simulink model "lineFollowerModel"  (R2020a)
settings: Solver=ode4  StartTime=0.0  StopTime=5  FixedStep=0.0001  RelTol=1e-3
values from neighbouring files (symbols this model uses):
  b = -0.05    [define_constants.m]
  cRoll = 0.1    [define_constants.m]
  g = 9.81    [define_constants.m]
  I_T = 0.1    [define_constants.m]
  I_yy = 5.0000e-05    (= 5e-05)    [define_constants.m]
  K = 0.0089    [define_constants.m]
  L = 2.3E-2    (= 0.023)    [define_constants.m]
  m_T = 1 * mass_scale    [define_constants.m]
  N = 50    [define_constants.m]
  R = Orientation    [GeoVerMakeCyl.m]    (also in define_constants.m = 2.2)
  row1 = 0.1    [define_constants.m]
  row2 = row1*wheel_ratio_scale    [define_constants.m]
  sX = row1    (= 0.1)    [define_constants.m]
  sY = 0    [define_constants.m]
  Vmax = 12    [define_constants.m]
  W = line_width/2    [define_constants.m]
  xLp = [(xL(1) - padamount*gridsize):gridsize:xL(1)-gridsize, xL, xL(end)+gridsize:gridsize:xL(end)+padamount*gridsize]    [define_constants.m]
  yLp = [(yL(1) - padamount*gridsize):gridsize:yL(1)-gridsize, yL, yL(end)+gridsize:gridsize:yL(end)+padamount*gridsize]    [define_constants.m]
  Z = zeros(dims)    [define_constants.m]
libraries: simulink x10
settings Model: Creator=Amir  LastModifiedBy=matthewterblanche
settings SFSimCC: CustomCodeUndefinedFunction=UseInterfaceOnly

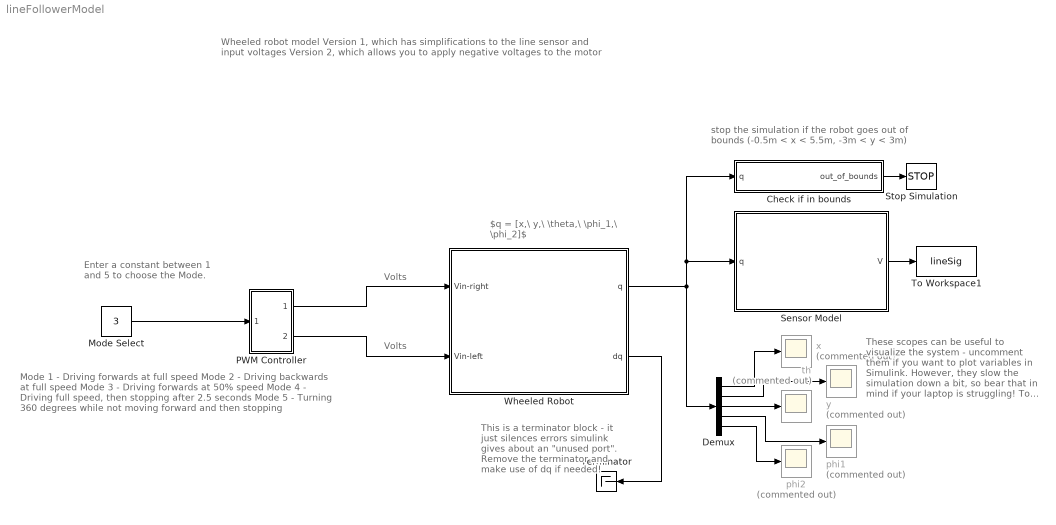
== system lineFollowerModel ==
  note: Volts
  note: stop the simulation if the robot goes out of bounds (-0.5m < x < 5.5m, -3m < y < 3m)
  note: Wheeled robot model
      | Version 1, which has simplifications to the line sensor and input voltages
      | Version 2, which allows you to apply negative voltages to the motor
  note: This is a terminator block - it just silences errors simulink gives about an "unused port". Remove the terminator and make use of dq if needed!
  note: These scopes can be useful to visualize the system - uncomment them if you want to plot variables in Simulink. However, they slow the simulation down a bit, so bear that in mind if your laptop is struggling!
      |
      | To make them work again, select the blocks > right click > Uncomment
  note: $q = [x,\ y,\ \theta,\ \phi_1,\ \phi_2]$
  note: Enter a constant between 1 and 5 to choose the Mode.
  note: Mode 1 - Driving forwards at full speed
      |
      | Mode 2 - Driving backwards at full speed
      |
      | Mode 3 - Driving forwards at 50% speed
      |
      | Mode 4 - Driving full speed, then stopping after 2.5 seconds
      |
      | Mode 5 - Turning 360 degrees while not moving forward and 			 then stopping
  note: Volts
  Check if in bounds : MATLAB Function  TreatAsAtomicUnit=on
  Demux : Demux  Outputs=5
  Mode Select : Constant  Value=3
  PWM Controller : Subsystem
  Sensor Model : Subsystem
  Stop Simulation : Stop
  Terminator : Terminator
  To Workspace1 : ToWorkspace  VariableName=lineSig  SampleTime=-1
  Wheeled Robot : Subsystem
  phi1 : Scope  Commented=on
  phi2 : Scope  Commented=on
  th : Scope  Commented=on
  x : Scope  Commented=on
  y : Scope  Commented=on
  wires:
  Demux/1 -> x/1
  Demux/2 -> y/1
  Demux/3 -> th/1
  Demux/4 -> phi1/1
  Demux/5 -> phi2/1
  Wheeled Robot/1(q) -> Sensor Model/1(q), Check if in bounds/1(q), Demux/1
  Sensor Model/1(V) -> To Workspace1/1
  Wheeled Robot/2(dq) -> Terminator/1
  Check if in bounds/1(out_of_bounds) -> Stop Simulation/1
  Mode Select/1 -> PWM Controller/1(In1)
  PWM Controller/1(Out1) -> Wheeled Robot/1(Vin-right)
  PWM Controller/2(Out2) -> Wheeled Robot/2(Vin-left)

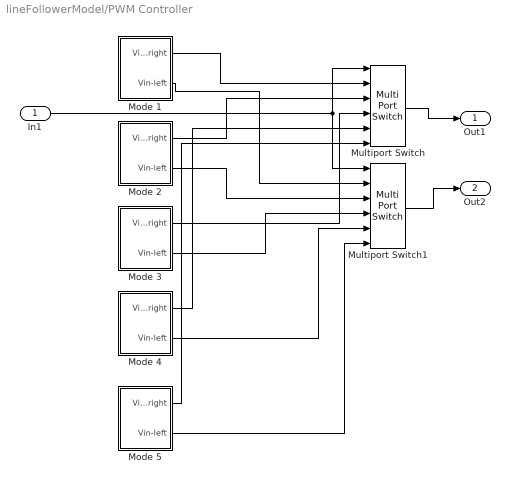
== system lineFollowerModel/PWM Controller ==
  In1 : Inport
  Mode 1 : Subsystem
  Mode 2 : Subsystem
  Mode 3 : Subsystem
  Mode 4 : Subsystem
  Mode 5 : Subsystem
  Multiport Switch : MultiPortSwitch  Inputs=5
  Multiport Switch1 : MultiPortSwitch  Inputs=5
  Out1 : Outport
  Out2 : Outport  Port=2
  wires:
  Multiport Switch/1 -> Out1/1
  Multiport Switch1/1 -> Out2/1
  In1/1 -> Multiport Switch/1, Multiport Switch1/1
  Mode 2/2(Vin-left) -> Multiport Switch1/3
  Mode 3/1(Vin-right) -> Multiport Switch/4
  Mode 5/2(Vin-left) -> Multiport Switch1/6
  Mode 4/1(Vin-right) -> Multiport Switch/5
  Mode 5/1(Vin-right) -> Multiport Switch/6
  Mode 2/1(Vin-right) -> Multiport Switch/3
  Mode 1/1(Vin-right) -> Multiport Switch/2
  Mode 1/2(Vin-left) -> Multiport Switch1/2
  Mode 4/2(Vin-left) -> Multiport Switch1/5
  Mode 3/2(Vin-left) -> Multiport Switch1/4

== system lineFollowerModel/Sensor Model ==
  q : Inport
  2-D Lookup Table : Lookup_n-D  BreakpointsForDimension1=xLp  BreakpointsForDimension2=yLp  Table=Z  InternalRulePriority=Speed  RndMeth=Simplest  InputSameDT=on
  MATLAB Function : MATLAB Function  TreatAsAtomicUnit=on
  V : Outport
  wires:
  MATLAB Function/1(posX) -> 2-D Lookup Table/1
  q/1 -> MATLAB Function/1(q)
  MATLAB Function/2(posY) -> 2-D Lookup Table/2
  2-D Lookup Table/1 -> V/1

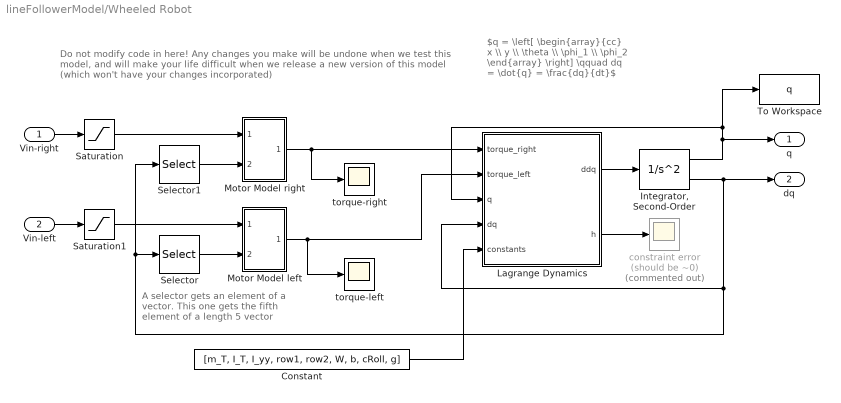
== system lineFollowerModel/Wheeled Robot ==
  note: A selector gets an element of a vector. This one gets the fifth element of a length 5 vector
  note: Do not modify code in here! Any changes you make will be undone when we test this model, and will make your life difficult when we release a new version of this model (which won't have your changes incorporated)
  note: $q = \left[ \begin{array}{cc} x \\ y \\ \theta \\ \phi_1 \\ \phi_2 \end{array} \right] \qquad dq = \dot{q} = \frac{dq}{dt}$
  Vin-right : Inport
  Vin-left : Inport  Port=2
  Constant : Constant  Value=[m_T, I_T, I_yy, row1, row2, W, b, cRoll, g]
  "Integrator, Second-Order" : SecondOrderIntegrator  ICX=[0 0 0 0 0]  ICDXDT=[0 0 0 0 0]
  Lagrange Dynamics : MATLAB Function  TreatAsAtomicUnit=on
  "Motor Model left " : Subsystem
  Motor Model right : Subsystem
  Saturation : Saturate  UpperLimit=Vmax  LowerLimit=-Vmax
  Saturation1 : Saturate  UpperLimit=Vmax  LowerLimit=-Vmax
  Selector : Selector  InputPortWidth=5  IndexOptions=Index vector (dialog)  Indices=[5]  OutputSizes=1
  Selector1 : Selector  InputPortWidth=5  IndexOptions=Index vector (dialog)  Indices=[4]  OutputSizes=1
  To Workspace : ToWorkspace  VariableName=q  SampleTime=0.01
  constraint error (should be ~0) : Scope  Commented=on
  torque-left : Scope
  torque-right : Scope
  q : Outport
  dq : Outport  Port=2
  wires:
  Selector/1 -> "Motor Model left "/2(Omega)
  Selector1/1 -> Motor Model right/2(Omega)
  Motor Model right/1(Tout) -> Lagrange Dynamics/1(torque_right), torque-right/1
  Vin-right/1 -> Saturation/1
  Vin-left/1 -> Saturation1/1
  "Integrator, Second-Order"/1 -> To Workspace/1, Lagrange Dynamics/3(q), q/1
  "Motor Model left "/1(Tout) -> Lagrange Dynamics/2(torque_left), torque-left/1
  "Integrator, Second-Order"/2 -> dq/1, Lagrange Dynamics/4(dq), Selector/1, Selector1/1
  Saturation/1 -> Motor Model right/1(Vin)
  Saturation1/1 -> "Motor Model left "/1(Vin)
  Lagrange Dynamics/1(ddq) -> "Integrator, Second-Order"/1
  Lagrange Dynamics/2(h) -> constraint error (should be ~0)/1
  Constant/1 -> Lagrange Dynamics/5(constants)

== system lineFollowerModel/PWM Controller/Mode 1 ==
  Subsystem : Subsystem
  Subsystem1 : Subsystem
  Vin-right : Outport
  Vin-left : Outport  Port=2
  wires:
  Subsystem1/1(Vin-left) -> Vin-left/1
  Subsystem/1(Vin-right) -> Vin-right/1

== system lineFollowerModel/PWM Controller/Mode 2 ==
  Subsystem : Subsystem
  Subsystem1 : Subsystem
  Vin-right : Outport
  Vin-left : Outport  Port=2
  wires:
  Subsystem1/1(Vin-left) -> Vin-left/1
  Subsystem/1(Vin-right) -> Vin-right/1

== system lineFollowerModel/PWM Controller/Mode 3 ==
  Subsystem : Subsystem
  Subsystem1 : Subsystem
  Vin-right : Outport
  Vin-left : Outport  Port=2
  wires:
  Subsystem1/1(Vin-left) -> Vin-left/1
  Subsystem/1(Vin-right) -> Vin-right/1

== system lineFollowerModel/PWM Controller/Mode 4 ==
  note: Stop motor after 2.5s
  Constant : Constant  Value=0
  Product : Product
  Product1 : Product
  Subsystem : Subsystem
  Subsystem1 : Subsystem
  Transport Delay : TransportDelay  DelayTime=2.5  InitialOutput=1  BufferSize=25600
  Vin-right : Outport
  Vin-left : Outport  Port=2
  wires:
  Subsystem1/1(Vin-left) -> Product/2
  Subsystem/1(Vin-right) -> Product1/2
  Product/1 -> Vin-left/1
  Product1/1 -> Vin-right/1
  Transport Delay/1 -> Product/1, Product1/1
  Constant/1 -> Transport Delay/1

== system lineFollowerModel/PWM Controller/Mode 5 ==
  Constant : Constant  Value=0
  Product : Product
  Product1 : Product
  Subsystem : Subsystem
  Subsystem1 : Subsystem
  Time motor must be on : TransportDelay  DelayTime=(0.175*pi/0.75)  InitialOutput=1  BufferSize=8192
  Vin-right : Outport
  Vin-left : Outport  Port=2
  wires:
  Constant/1 -> Time motor must be on/1
  Time motor must be on/1 -> Product1/1, Product/1
  Subsystem/1(Vin-right) -> Product/2
  Product/1 -> Vin-right/1
  Subsystem1/1(Vin-left) -> Product1/2
  Product1/1 -> Vin-left/1

== system lineFollowerModel/Wheeled Robot/Motor Model left  ==
  Vin : Inport
  Omega : Inport  Port=2
  Integrator : Integrator
  KT : Gain  Gain=K
  current dynamics : MATLAB Function  TreatAsAtomicUnit=on
  gear : Gain  Gain=N
  gear1 : Gain  Gain=N
  Tout : Outport  VectorParamsAs1DForOutWhenUnconnected=off
  wires:
  gear1/1 -> current dynamics/3(dth)
  Integrator/1 -> current dynamics/2(i), KT/1
  Omega/1 -> gear1/1
  gear/1 -> Tout/1
  current dynamics/1(di) -> Integrator/1
  KT/1 -> gear/1
  Vin/1 -> current dynamics/1(V)

== system lineFollowerModel/Wheeled Robot/Motor Model right ==
  Vin : Inport
  Omega : Inport  Port=2
  Integrator : Integrator
  KT : Gain  Gain=K
  current dynamics : MATLAB Function  TreatAsAtomicUnit=on
  gear : Gain  Gain=N
  gear1 : Gain  Gain=N
  Tout : Outport  VectorParamsAs1DForOutWhenUnconnected=off
  wires:
  Vin/1 -> current dynamics/1(V)
  KT/1 -> gear/1
  current dynamics/1(di) -> Integrator/1
  gear/1 -> Tout/1
  Omega/1 -> gear1/1
  Integrator/1 -> current dynamics/2(i), KT/1
  gear1/1 -> current dynamics/3(dth)

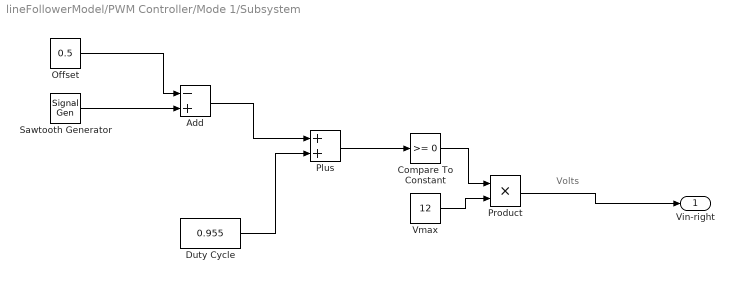
== system lineFollowerModel/PWM Controller/Mode 1/Subsystem ==
  note: Volts
  Add : Sum  Inputs=-+
  Compare To Constant : simulink/Logic and Bit Operations/Compare To Constant  relop=>=  const=0  OutDataTypeStr=boolean
  Duty Cycle : Constant  Value=0.955
  Offset : Constant  Value=0.5
  Plus : Sum
  Product : Product
  Sawtooth Generator : SignalGenerator  WaveForm=sawtooth  Amplitude=0.5  Frequency=10
  Vmax : Constant  Value=12
  Vin-right : Outport
  wires:
  Sawtooth Generator/1 -> Add/2
  Product/1 -> Vin-right/1
  Vmax/1 -> Product/2
  Duty Cycle/1 -> Plus/2
  Plus/1 -> Compare To Constant/1
  Offset/1 -> Add/1
  Compare To Constant/1 -> Product/1
  Add/1 -> Plus/1

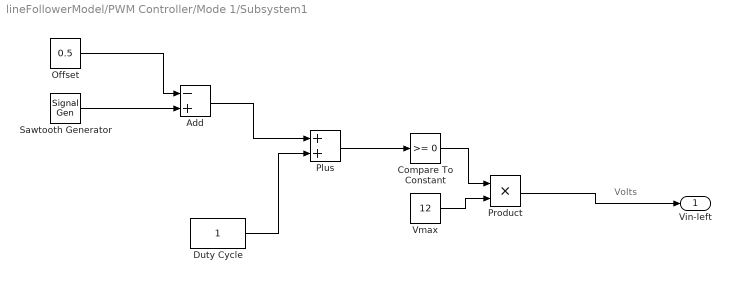
== system lineFollowerModel/PWM Controller/Mode 1/Subsystem1 ==
  note: Volts
  Add : Sum  Inputs=-+
  Compare To Constant : simulink/Logic and Bit Operations/Compare To Constant  relop=>=  const=0  OutDataTypeStr=boolean
  Duty Cycle : Constant
  Offset : Constant  Value=0.5
  Plus : Sum
  Product : Product
  Sawtooth Generator : SignalGenerator  WaveForm=sawtooth  Amplitude=0.5  Frequency=10
  Vmax : Constant  Value=12
  Vin-left : Outport
  wires:
  Sawtooth Generator/1 -> Add/2
  Product/1 -> Vin-left/1
  Vmax/1 -> Product/2
  Duty Cycle/1 -> Plus/2
  Plus/1 -> Compare To Constant/1
  Offset/1 -> Add/1
  Compare To Constant/1 -> Product/1
  Add/1 -> Plus/1

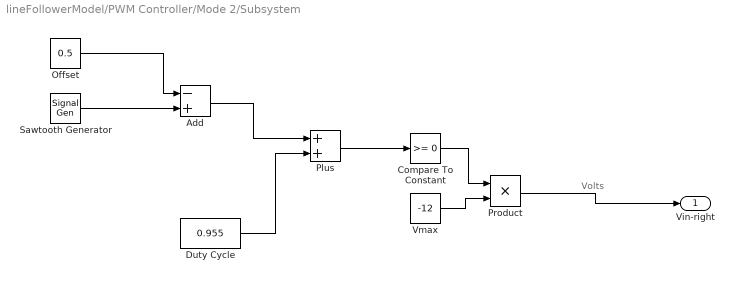
== system lineFollowerModel/PWM Controller/Mode 2/Subsystem ==
  note: Volts
  Add : Sum  Inputs=-+
  Compare To Constant : simulink/Logic and Bit Operations/Compare To Constant  relop=>=  const=0  OutDataTypeStr=boolean
  Duty Cycle : Constant  Value=0.955
  Offset : Constant  Value=0.5
  Plus : Sum
  Product : Product
  Sawtooth Generator : SignalGenerator  WaveForm=sawtooth  Amplitude=0.5  Frequency=10
  Vmax : Constant  Value=-12
  Vin-right : Outport
  wires:
  Sawtooth Generator/1 -> Add/2
  Product/1 -> Vin-right/1
  Vmax/1 -> Product/2
  Duty Cycle/1 -> Plus/2
  Plus/1 -> Compare To Constant/1
  Offset/1 -> Add/1
  Compare To Constant/1 -> Product/1
  Add/1 -> Plus/1

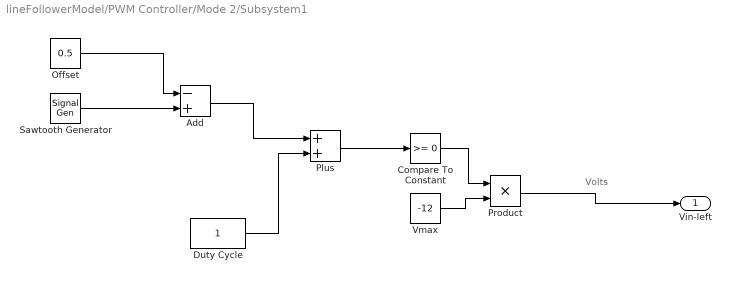
== system lineFollowerModel/PWM Controller/Mode 2/Subsystem1 ==
  note: Volts
  Add : Sum  Inputs=-+
  Compare To Constant : simulink/Logic and Bit Operations/Compare To Constant  relop=>=  const=0  OutDataTypeStr=boolean
  Duty Cycle : Constant
  Offset : Constant  Value=0.5
  Plus : Sum
  Product : Product
  Sawtooth Generator : SignalGenerator  WaveForm=sawtooth  Amplitude=0.5  Frequency=10
  Vmax : Constant  Value=-12
  Vin-left : Outport
  wires:
  Sawtooth Generator/1 -> Add/2
  Product/1 -> Vin-left/1
  Vmax/1 -> Product/2
  Duty Cycle/1 -> Plus/2
  Plus/1 -> Compare To Constant/1
  Offset/1 -> Add/1
  Compare To Constant/1 -> Product/1
  Add/1 -> Plus/1

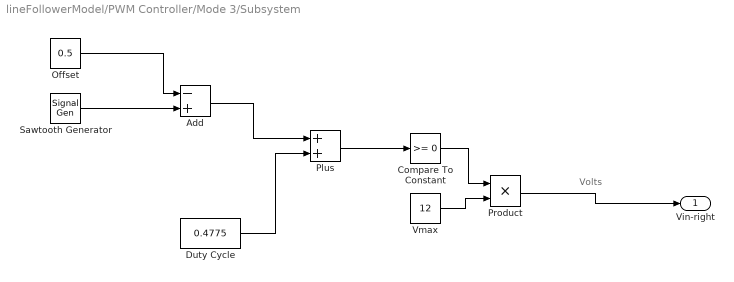
== system lineFollowerModel/PWM Controller/Mode 3/Subsystem ==
  note: Volts
  Add : Sum  Inputs=-+
  Compare To Constant : simulink/Logic and Bit Operations/Compare To Constant  relop=>=  const=0  OutDataTypeStr=boolean
  Duty Cycle : Constant  Value=0.4775
  Offset : Constant  Value=0.5
  Plus : Sum
  Product : Product
  Sawtooth Generator : SignalGenerator  WaveForm=sawtooth  Amplitude=0.5  Frequency=10
  Vmax : Constant  Value=12
  Vin-right : Outport
  wires:
  Sawtooth Generator/1 -> Add/2
  Product/1 -> Vin-right/1
  Vmax/1 -> Product/2
  Duty Cycle/1 -> Plus/2
  Plus/1 -> Compare To Constant/1
  Offset/1 -> Add/1
  Compare To Constant/1 -> Product/1
  Add/1 -> Plus/1

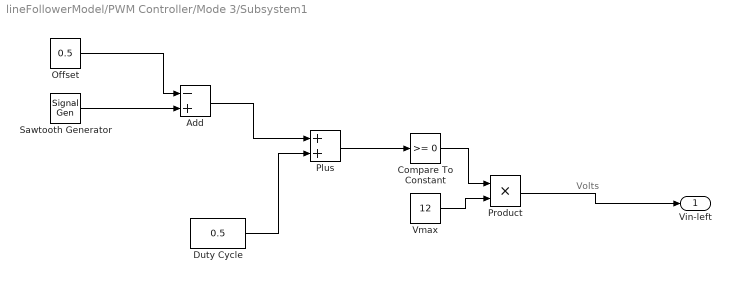
== system lineFollowerModel/PWM Controller/Mode 3/Subsystem1 ==
  note: Volts
  Add : Sum  Inputs=-+
  Compare To Constant : simulink/Logic and Bit Operations/Compare To Constant  relop=>=  const=0  OutDataTypeStr=boolean
  Duty Cycle : Constant  Value=0.5
  Offset : Constant  Value=0.5
  Plus : Sum
  Product : Product
  Sawtooth Generator : SignalGenerator  WaveForm=sawtooth  Amplitude=0.5  Frequency=10
  Vmax : Constant  Value=12
  Vin-left : Outport
  wires:
  Sawtooth Generator/1 -> Add/2
  Product/1 -> Vin-left/1
  Vmax/1 -> Product/2
  Duty Cycle/1 -> Plus/2
  Plus/1 -> Compare To Constant/1
  Offset/1 -> Add/1
  Compare To Constant/1 -> Product/1
  Add/1 -> Plus/1

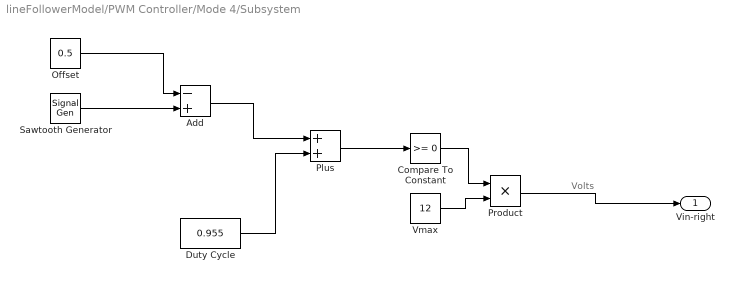
== system lineFollowerModel/PWM Controller/Mode 4/Subsystem ==
  note: Volts
  Add : Sum  Inputs=-+
  Compare To Constant : simulink/Logic and Bit Operations/Compare To Constant  relop=>=  const=0  OutDataTypeStr=boolean
  Duty Cycle : Constant  Value=0.955
  Offset : Constant  Value=0.5
  Plus : Sum
  Product : Product
  Sawtooth Generator : SignalGenerator  WaveForm=sawtooth  Amplitude=0.5  Frequency=10
  Vmax : Constant  Value=12
  Vin-right : Outport
  wires:
  Sawtooth Generator/1 -> Add/2
  Product/1 -> Vin-right/1
  Vmax/1 -> Product/2
  Duty Cycle/1 -> Plus/2
  Plus/1 -> Compare To Constant/1
  Offset/1 -> Add/1
  Compare To Constant/1 -> Product/1
  Add/1 -> Plus/1

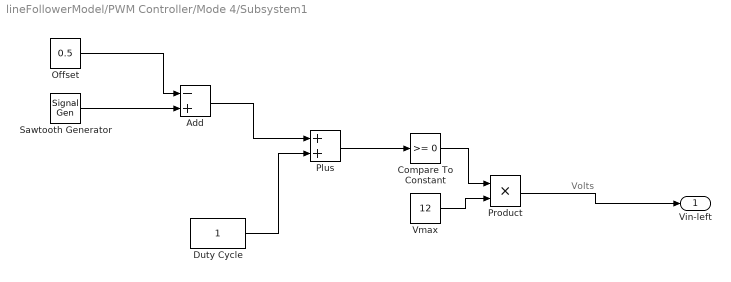
== system lineFollowerModel/PWM Controller/Mode 4/Subsystem1 ==
  note: Volts
  Add : Sum  Inputs=-+
  Compare To Constant : simulink/Logic and Bit Operations/Compare To Constant  relop=>=  const=0  OutDataTypeStr=boolean
  Duty Cycle : Constant
  Offset : Constant  Value=0.5
  Plus : Sum
  Product : Product
  Sawtooth Generator : SignalGenerator  WaveForm=sawtooth  Amplitude=0.5  Frequency=10
  Vmax : Constant  Value=12
  Vin-left : Outport
  wires:
  Sawtooth Generator/1 -> Add/2
  Product/1 -> Vin-left/1
  Vmax/1 -> Product/2
  Duty Cycle/1 -> Plus/2
  Plus/1 -> Compare To Constant/1
  Offset/1 -> Add/1
  Compare To Constant/1 -> Product/1
  Add/1 -> Plus/1

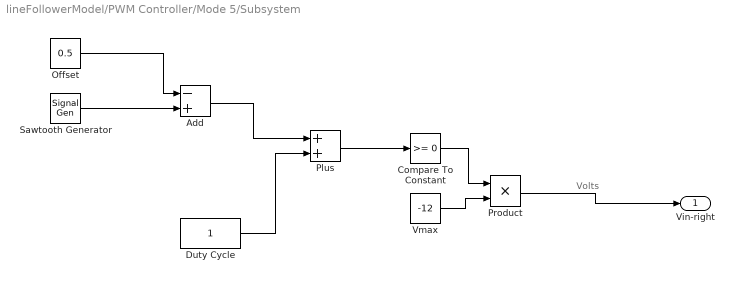
== system lineFollowerModel/PWM Controller/Mode 5/Subsystem ==
  note: Volts
  Add : Sum  Inputs=-+
  Compare To Constant : simulink/Logic and Bit Operations/Compare To Constant  relop=>=  const=0  OutDataTypeStr=boolean
  Duty Cycle : Constant
  Offset : Constant  Value=0.5
  Plus : Sum
  Product : Product
  Sawtooth Generator : SignalGenerator  WaveForm=sawtooth  Amplitude=0.5  Frequency=10
  Vmax : Constant  Value=-12
  Vin-right : Outport
  wires:
  Sawtooth Generator/1 -> Add/2
  Product/1 -> Vin-right/1
  Vmax/1 -> Product/2
  Duty Cycle/1 -> Plus/2
  Plus/1 -> Compare To Constant/1
  Offset/1 -> Add/1
  Compare To Constant/1 -> Product/1
  Add/1 -> Plus/1

== system lineFollowerModel/PWM Controller/Mode 5/Subsystem1 ==
  note: Volts
  Add : Sum  Inputs=-+
  Compare To Constant : simulink/Logic and Bit Operations/Compare To Constant  relop=>=  const=0  OutDataTypeStr=boolean
  Duty Cycle : Constant  Value=0.9
  Offset : Constant  Value=0.5
  Plus : Sum
  Product : Product
  Sawtooth Generator : SignalGenerator  WaveForm=sawtooth  Amplitude=0.5  Frequency=10
  Vmax : Constant  Value=12
  Vin-left : Outport
  wires:
  Sawtooth Generator/1 -> Add/2
  Product/1 -> Vin-left/1
  Vmax/1 -> Product/2
  Duty Cycle/1 -> Plus/2
  Plus/1 -> Compare To Constant/1
  Offset/1 -> Add/1
  Compare To Constant/1 -> Product/1
  Add/1 -> Plus/1

== matlab function lineFollowerModel/Wheeled Robot/Motor Model left /current dynamics ==
  data: V input; di output; i input; L parameter; K parameter; R parameter; dth input
function di = dyn(V, i, L, K, R, dth)

di = (V-K*dth-R*i)/L;

== matlab function lineFollowerModel/Wheeled Robot/Lagrange Dynamics ==
  settings: updateMethod=DISCRETE
  data: ddq output size=5; h output size=3; torque_right input; torque_left input; q input; dq input; constants input
%% These dynamics are based on: 
% https://robotics.caltech.edu/~me72/class/DiffDrive2.pdf
% Assume 'd' is 0
function [ddq, h] = dyn(torque_right, torque_left, q, dq, constants)
m_T = constants(1);
I_T = constants(2);
I_yy = constants(3);
row1 = constants(4);
row2 = constants(5);
W = constants(6);
b = constants(7);
cRoll = constants(8);
g = constants(9);

%% Admin
% x = q(1);
% y = q(2);
th = q(3);
% phi1 = q(4);
% phi2 = q(5);

dx = dq(1);
dy = dq(2);
dth = dq(3);
dphi1 = dq(4);
dphi2 = dq(5);


%% Calculate the matrices
% Mass
M = [m_T,   0,   0,    0,    0
       0, m_T,   0,    0,    0
       0,   0, I_T,    0,    0
       0,   0,   0, I_yy,    0
       0,   0,   0,    0, I_yy];

temp = [-sin(th), cos(th), cos(th)
         cos(th), sin(th), sin(th)
               0,     W/2,    -W/2
               0,  - row1,       0
               0,       0,   -row2];

C = transpose(temp);

temp = [ -dth*cos(th), -dth*sin(th), -dth*sin(th)
         -dth*sin(th),  dth*cos(th),  dth*cos(th)
                    0,            0,            0
                    0,            0,            0
                    0,            0,            0];

dC = transpose(temp);

% Input force
T = [0; 0; 0; torque_right + b*dphi1; torque_left + b*dphi2];

% Rolling resistance
vWheel1 = (W*dth)/2 + dx*cos(th) + dy*sin(th);
vWheel2 = dx*cos(th) - (W*dth)/2 + dy*sin(th);
sgnWheel1 = sign(vWheel1);
sgnWheel2 = sign(vWheel2);

F1 = -sgnWheel1*m_T*g*cRoll;
F2 = -sgnWheel2*m_T*g*cRoll;

% input force mapping
Q =  [F1*cos(th) + F2*cos(th)
      F1*sin(th) + F2*sin(th)
          (F1*W)/2 - (F2*W)/2
                            0
                            0];

%% Calculate Lagrange Multipliers
% lambda = -inv(C*inv(M)*transpose(C))*(C*inv(M)*(T+Q) + dC*dq);
lambda = -inv(C*(M\transpose(C)))*(C*(M\(T+Q)) + dC*dq);

h = [                          dy*cos(th) - dx*sin(th)
      (W*dth)/2 - dphi1*row1 + dx*cos(th) + dy*sin(th)
      dx*cos(th) - dphi2*row2 - (W*dth)/2 + dy*sin(th)];


%% Calculate acceleration
ddq = M\(transpose(C)*lambda + T + Q);

end

== matlab function lineFollowerModel/Wheeled Robot/Motor Model right/current dynamics ==
  data: V input; di output; i input; L parameter; K parameter; R parameter; dth input
function di = dyn(V, i, L, K, R, dth)

di = (V - K*dth - R*i)/L;

== matlab function lineFollowerModel/Sensor Model/MATLAB Function ==
  data: posX output; q input; sY parameter; sX parameter; posY output
function [posX, posY] = sensorPosition(q, sY, sX)

x = q(1);
y = q(2);
th = q(3);

% Position of sensor in inertial
posSens_I = [x + sX*cos(th) - sY*sin(th)
             y + sY*cos(th) + sX*sin(th)];

posX = posSens_I(1);
posY = posSens_I(2);

== matlab function lineFollowerModel/Check if in bounds ==
  data: q input; out_of_bounds output
function out_of_bounds = fcn(q)
x = q(1);
y = q(2);

in_bounds = -0.5 < x && x < 5.5 && -3 < y && y < 3;

out_of_bounds = ~in_bounds;

if out_of_bounds
    disp("Stopping simulation - robot is out of bounds!")
end
